simulink library "INT_EngDa_PwrEng"  (R2016b)
settings: Solver=VariableStepAuto  StartTime=0.0  StopTime=10.0  RelTol=1e-3
settings Model: Creator=Administrator  LastModifiedBy=Administrator

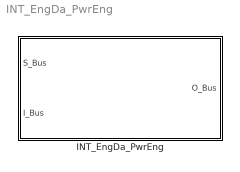
== system INT_EngDa_PwrEng ==
  INT_EngDa_PwrEng : Subsystem

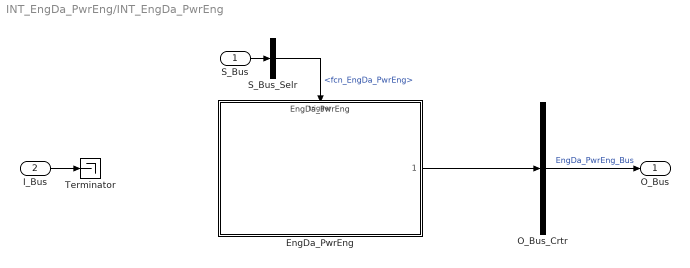
== system INT_EngDa_PwrEng/INT_EngDa_PwrEng ==
  S_Bus : Inport
  I_Bus : Inport  Port=2
  EngDa_PwrEng : ModelReference  ModelNameDialog=EngDa_PwrEng  SimulationMode=Normal  ModelReferenceVersion=1.2  TriggerPortName=function  TriggerPortTriggerType=function-call  TriggerPortStatesWhenEnabling=held
  O_Bus_Crtr : BusCreator  Inputs=1
  S_Bus_Selr : BusSelector  OutputSignals=fcn_EngDa_PwrEng
  Terminator : Terminator
  O_Bus : Outport
  wires:
  S_Bus_Selr/1 -> EngDa_PwrEng/Trigger  "<fcn_EngDa_PwrEng>"
  S_Bus/1 -> S_Bus_Selr/1
  I_Bus/1 -> Terminator/1
  O_Bus_Crtr/1 -> O_Bus/1  "EngDa_PwrEng_Bus"
  EngDa_PwrEng/1 -> O_Bus_Crtr/1
